simulink model "RainSnsrWiperMot_Method_2"  (R2021b)
settings: Solver=FixedStepDiscrete  StartTime=0.0  StopTime=20  FixedStep=0.01  RelTol=1e-3
model workspace (MAT data in the model file):
  Table_x_data = Simulink.Parameter
  Table_x_data.Value = [0 1 2 3 4 5 6 7]
  Table_x_data.DataType = 'auto'
  Table_x_data.Complexity = 'real'
  Table_x_data.Dimensions = [1 8]
  Table_y_data = Simulink.Parameter
  Table_y_data.Value = [0 0.4 0.45 0.5 0.55 0.6 0.65 0.7]
  Table_y_data.DataType = 'auto'
  Table_y_data.Complexity = 'real'
  Table_y_data.Dimensions = [1 8]
undefined symbols (not defined in the file or in its folder): sigbuilder_block
libraries: simulink x2
settings Model: Creator=waleed.elshemy  LastModifiedBy=waleed.elshemy
settings OptimizationCC: DefaultParameterBehavior=Inlined  UseDivisionForNetSlopeComputation=on  GainParamInheritBuiltInType=on  UseFloatMulNetSlope=on  InlineInvariantSignals=on  PassReuseOutputArgsAs=Individual arguments  ZeroExternalMemoryAtStartup=off  ZeroInternalMemoryAtStartup=off  NoFixptDivByZeroProtection=on  EfficientFloat2IntCast=on  LifeSpan=1  OptimizeBlockOrder=speed  DifferentSizesBufferReuse=on  EfficientTunableParamExpr=on
settings DebuggingCC: ParameterTunabilityLossMsg=error
settings HardwareCC: ProdLongLongMode=on
settings SFSimCC: MATLABDynamicMemAlloc=off
settings RTWCC: Description=Embedded Coder  SystemTargetFile=ert.tlc  TemplateMakefile=ert_default_tmf
settings CodeAppCC: ForceParamTrailComments=on  IgnoreCustomStorageClasses=off  OperatorAnnotations=on  SimulinkDataObjDesc=on  SFDataObjDesc=on  CustomSymbolStrGlobalVar=rt$N$M  CustomSymbolStrType=$N$M  CustomSymbolStrFcn=$N$M$F  CustomSymbolStrMacro=$N$M  InsertBlockDesc=on
settings ERTTargetCC: TargetLangStandard=C99 (ISO)  GenerateSampleERTMain=on  IncludeMdlTerminateFcn=off  CombineSignalStateStructs=on  SupportComplex=off  SupportNonInlinedSFcns=on  InlinedParameterPlacement=NonHierarchical  ERTCustomFileTemplate=example_file_process.tlc  ERTFilePackagingFormat=CompactWithDataFile

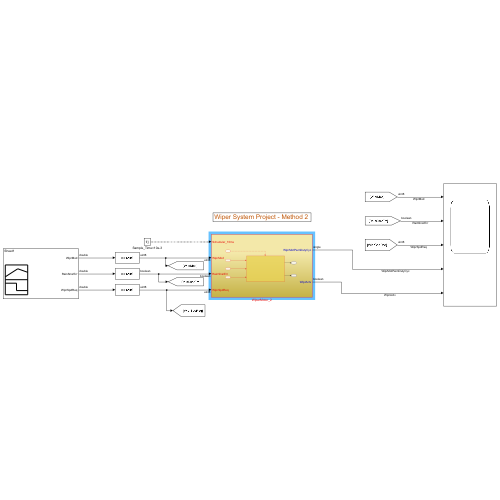
[thumbnail: Simulink's stored preview of the top-level diagram]
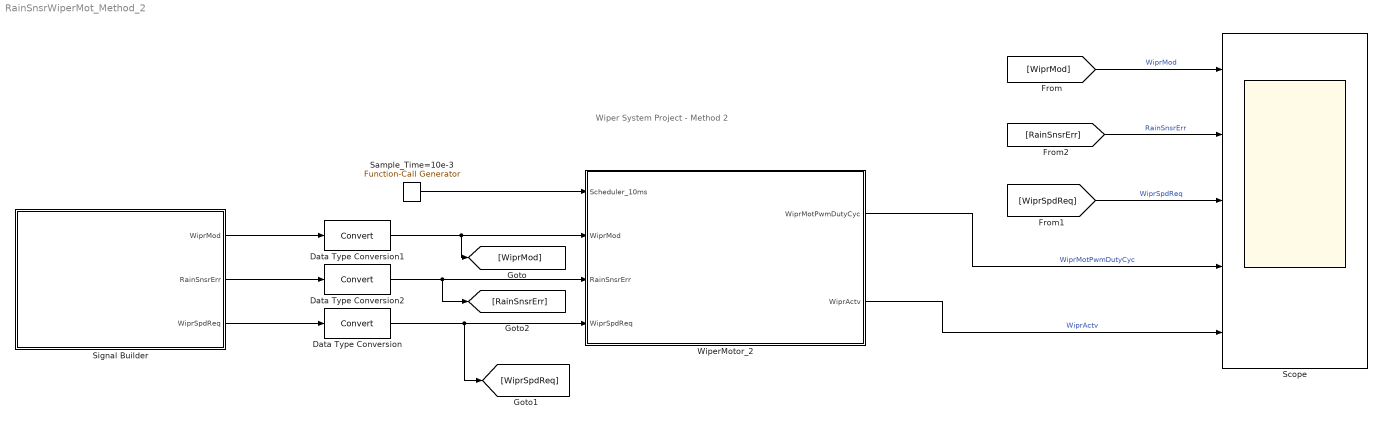
== system RainSnsrWiperMot_Method_2 ==
  note: Wiper System Project - Method 2
  Data Type Conversion : DataTypeConversion
  Data Type Conversion1 : DataTypeConversion
  Data Type Conversion2 : DataTypeConversion
  Sample_Time=10e-3 : simulink/Ports & Subsystems/Function-Call Generator  sample_time=0.01  numberOfIterations=1  DisallowWideOutput=off
  Scope : Scope  NumInputPorts=5
  Signal Builder : Subsystem  Tag=STV Subsys  LoadFcn=sigbuilder_block('load');  StartFcn=sigbuilder_block('start');  StopFcn=sigbuilder_block('stop');  ClipboardFcn=sigbuilder_block('clipboard');  mask(Sigbuilder block){tuvar=[0:10]}
      mask help: Simulink:masks:SigbuilderBlock_MD
      mask init:
      | if ~strcmp(get_param(bdroot(gcbh),'SimulationStatus'),'stopped') tuvar = sigbuilder_block('maskInit'); end
      settings: CopyFcn=sigbuilder_block('copy');  DeleteFcn=sigbuilder_block('delete');  ModelCloseFcn=sigbuilder_block('modelClose');  PreSaveFcn=sigbuilder_block('preSave');  PauseFcn=sigbuilder_block('pause');  ContinueFcn=sigbuilder_block('continue');  NameChangeFcn=sigbuilder_block('namechange');  OpenFcn=sigbuilder_block('open',[240 92.5 550.5 362.5 ]);  CloseFcn=sigbuilder_block('close');
      mask Display: plot(0, 0, 100, 100,[2, 2, 32, 32, 2], [68, 8, 8, 68, 68],[32, 2], [38, 38], [32, 19, 2],[53, 60, 44], [32, 17, 17, 2],[16, 16, 31, 31]);txt = getActiveGroup(gcbh);text(2, 100, txt,'verticalAlignment', 'top');
  WiperMotor_2 : Subsystem
  wires:
  Sample_Time=10e-3/1 -> WiperMotor_2/1(Scheduler_10ms)
  WiperMotor_2/1(WiprMotPwmDutyCyc) -> Scope/4  "WiprMotPwmDutyCyc"
  WiperMotor_2/2(WiprActv) -> Scope/5  "WiprActv"
  Signal Builder/1(WiprMod) -> Data Type Conversion1/1
  Signal Builder/2(RainSnsrErr) -> Data Type Conversion2/1
  Signal Builder/3(WiprSpdReq) -> Data Type Conversion/1
  Data Type Conversion/1 -> WiperMotor_2/4(WiprSpdReq), [WiprSpdReq]
  Data Type Conversion1/1 -> WiperMotor_2/2(WiprMod), [WiprMod]
  [WiprMod] -> Scope/1  "WiprMod"
  [WiprSpdReq] -> Scope/3  "WiprSpdReq"
  [RainSnsrErr] -> Scope/2  "RainSnsrErr"
  Data Type Conversion2/1 -> [RainSnsrErr], WiperMotor_2/3(RainSnsrErr)

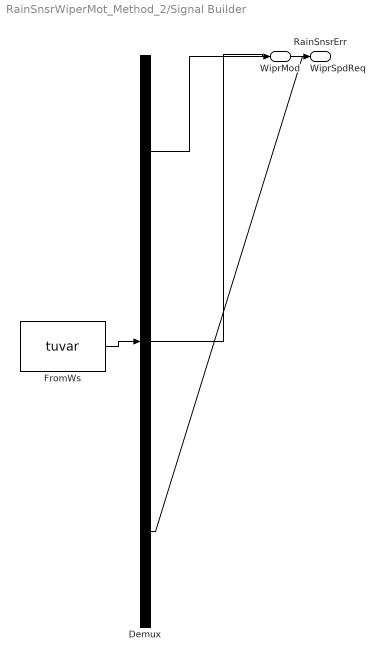
== system RainSnsrWiperMot_Method_2/Signal Builder ==
  Demux : Demux  Tag=STV Demux  Outputs=3
      settings: DisplayOption=none
  FromWs : FromWorkspace  Tag=STV FromWs  VariableName=tuvar  SampleTime=1  OutputAfterFinalValue=Holding final value
      SigBuilderData=|
      | common.afterFinalStr = 'Hold final value'
      | common.sampleTime = '1'
      | dataSet.timeRange = [0 16]
      | dataSet.name = 'Sheet1'
      | sbobj.Groups.Name = 'Sheet1'
      | sbobj.Groups.Signals(1).Name = 'WiprMod'
      | sbobj.Groups.Signals(1).XData = [0 1 2 3 4 5 6 7 8 9 10 11 12 13 14 15 16]
      | sbobj.Groups.Signals(1).YData = [0 0 2 2 3 3 1 1 1 1 1 1 1 1 1 1 1]
      | sbobj.Groups.Signals(2).Name = 'RainSnsrErr'
      | sbobj.Groups.Signals(2).XData = [0 1 2 3 4 5 6 7 8 9 10 11 12 13 14 15 16]
      | sbobj.Groups.Signals(2).YData = [0 0 0 0 0 0 0 0 0 0 0 0 0 0 0 1 0]
      | sbobj.Groups.Signals(3).Name = 'WiprSpdReq'
      | sbobj.Groups.Signals(3).XData = [0 1 2 3 4 5 6 7 8 9 10 11 12 13 14 15 16]
      | sbobj.Groups.Signals(3).YData = [0 0 0 0 0 0 0 0 1 2 3 4 5 6 7 7 7]
      | sbobj.Groups.TimeRange = [0 16]
  WiprMod : Outport  Tag=STV Outport
  RainSnsrErr : Outport  Tag=STV Outport  Port=2
  WiprSpdReq : Outport  Tag=STV Outport  Port=3
  wires:
  Demux/1 -> WiprMod/1
  FromWs/1 -> Demux/1
  Demux/2 -> RainSnsrErr/1
  Demux/3 -> WiprSpdReq/1

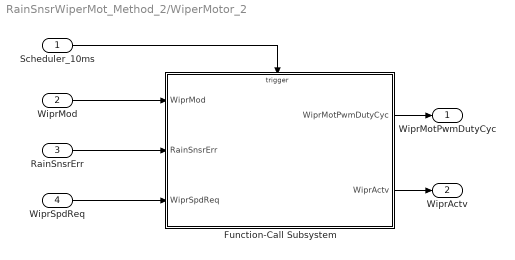
== system RainSnsrWiperMot_Method_2/WiperMotor_2 ==
  Scheduler_10ms : Inport
  WiprMod : Inport  Port=2  OutMin=0  OutMax=3  OutDataTypeStr=uint8
  RainSnsrErr : Inport  Port=3  OutMin=0  OutMax=1  OutDataTypeStr=boolean
  WiprSpdReq : Inport  Port=4  OutMin=0  OutMax=7  OutDataTypeStr=uint8
  Function-Call Subsystem : Subsystem  TreatAsAtomicUnit=on
  WiprMotPwmDutyCyc : Outport  OutMin=0  OutMax=1  OutDataTypeStr=single  LockScale=on
  WiprActv : Outport  Port=2  OutDataTypeStr=boolean
  wires:
  WiprMod/1 -> Function-Call Subsystem/1(WiprMod)
  WiprSpdReq/1 -> Function-Call Subsystem/3(WiprSpdReq)
  Function-Call Subsystem/2(WiprActv) -> WiprActv/1
  Scheduler_10ms/1 -> Function-Call Subsystem/Trigger
  RainSnsrErr/1 -> Function-Call Subsystem/2(RainSnsrErr)
  Function-Call Subsystem/1(WiprMotPwmDutyCyc) -> WiprMotPwmDutyCyc/1

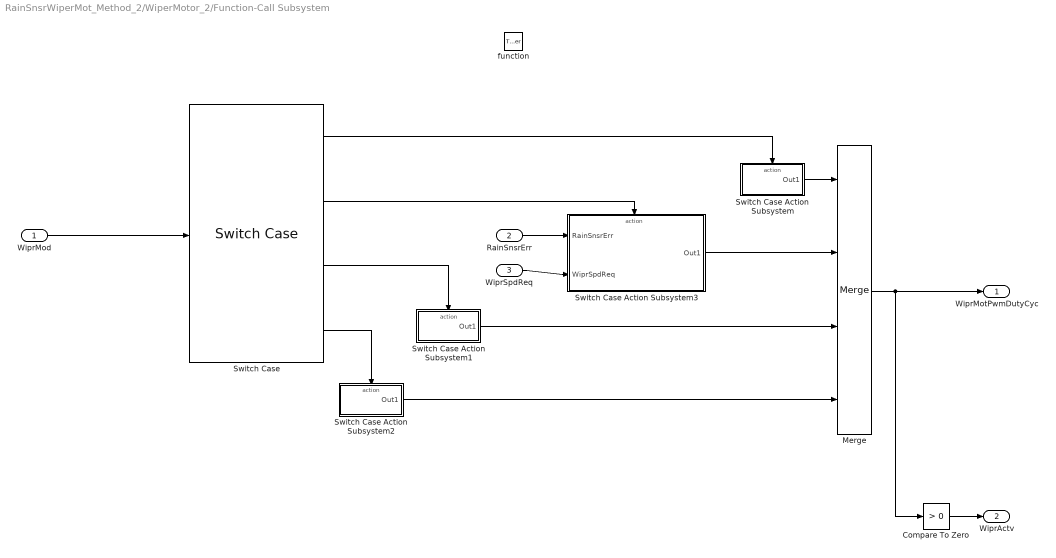
== system RainSnsrWiperMot_Method_2/WiperMotor_2/Function-Call Subsystem ==
  WiprMod : Inport
  RainSnsrErr : Inport  Port=2
  WiprSpdReq : Inport  Port=3
  function : TriggerPort  TriggerType=function-call  VariantControl=(inherit)
  Compare To Zero : simulink/Logic and Bit Operations/Compare To Zero  relop=>  OutDataTypeStr=boolean
  Merge : Merge  Inputs=4
  Switch Case : SwitchCase  CaseConditions={0,1,2,3}  ShowDefaultCase=off
  Switch Case Action Subsystem : Subsystem  TreatAsAtomicUnit=on
  Switch Case Action Subsystem1 : Subsystem  TreatAsAtomicUnit=on
  Switch Case Action Subsystem2 : Subsystem  TreatAsAtomicUnit=on
  Switch Case Action Subsystem3 : Subsystem  TreatAsAtomicUnit=on
  WiprMotPwmDutyCyc : Outport
  WiprActv : Outport  Port=2
  wires:
  WiprMod/1 -> Switch Case/1
  Switch Case/4 -> Switch Case Action Subsystem2/Action
  Switch Case/1 -> Switch Case Action Subsystem/Action
  Switch Case/2 -> Switch Case Action Subsystem3/Action
  Switch Case/3 -> Switch Case Action Subsystem1/Action
  Switch Case Action Subsystem/1(Out1) -> Merge/1
  Switch Case Action Subsystem3/1(Out1) -> Merge/2
  Switch Case Action Subsystem1/1(Out1) -> Merge/3
  Switch Case Action Subsystem2/1(Out1) -> Merge/4
  RainSnsrErr/1 -> Switch Case Action Subsystem3/1(RainSnsrErr)
  WiprSpdReq/1 -> Switch Case Action Subsystem3/2(WiprSpdReq)
  Merge/1 -> Compare To Zero/1, WiprMotPwmDutyCyc/1
  Compare To Zero/1 -> WiprActv/1

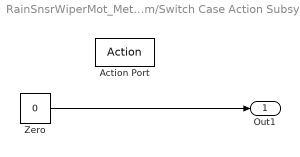
== system RainSnsrWiperMot_Method_2/WiperMotor_2/Function-Call Subsystem/Switch Case Action Subsystem ==
  Action Port : ActionPort  ActionPortLabel=case [ 0 ]:
  Zero : Constant  Value=0  OutDataTypeStr=Inherit: Inherit via back propagation
  Out1 : Outport
  wires:
  Zero/1 -> Out1/1

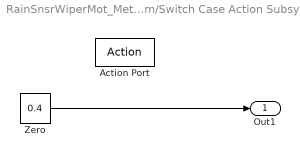
== system RainSnsrWiperMot_Method_2/WiperMotor_2/Function-Call Subsystem/Switch Case Action Subsystem1 ==
  Action Port : ActionPort  ActionPortLabel=case [ 2 ]:
  Zero : Constant  Value=0.4  OutDataTypeStr=single
  Out1 : Outport
  wires:
  Zero/1 -> Out1/1

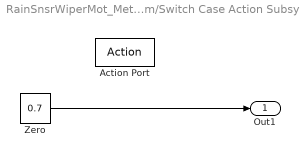
== system RainSnsrWiperMot_Method_2/WiperMotor_2/Function-Call Subsystem/Switch Case Action Subsystem2 ==
  Action Port : ActionPort  ActionPortLabel=case [ 3 ]:
  Zero : Constant  Value=0.7  OutDataTypeStr=Inherit: Inherit via back propagation
  Out1 : Outport
  wires:
  Zero/1 -> Out1/1

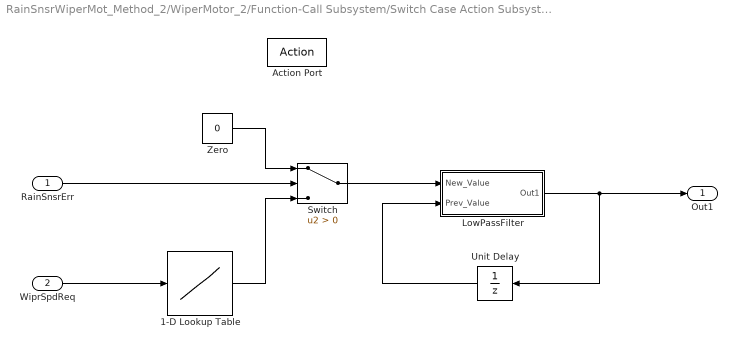
== system RainSnsrWiperMot_Method_2/WiperMotor_2/Function-Call Subsystem/Switch Case Action Subsystem3 ==
  RainSnsrErr : Inport
  WiprSpdReq : Inport  Port=2
  Action Port : ActionPort  ActionPortLabel=case [ 1 ]:
  1-D Lookup Table : Lookup_n-D  NumberOfTableDimensions=1  BreakpointsForDimension1=Table_x_data  Table=Table_y_data  TableDataTypeStr=single  ExtrapMethod=Clip  InternalRulePriority=Speed  OutDataTypeStr=single  RndMeth=Simplest  InputSameDT=on
  LowPassFilter : Subsystem
  Switch : Switch  Criteria=u2 > Threshold
  Unit Delay : UnitDelay  SampleTime=-1  HasFrameUpgradeWarning=on
  Zero : Constant  Value=0  OutDataTypeStr=Inherit: Inherit via back propagation
  Out1 : Outport
  wires:
  RainSnsrErr/1 -> Switch/2
  Zero/1 -> Switch/1
  WiprSpdReq/1 -> 1-D Lookup Table/1
  1-D Lookup Table/1 -> Switch/3
  Switch/1 -> LowPassFilter/1(New_Value)
  Unit Delay/1 -> LowPassFilter/2(Prev_Value)
  LowPassFilter/1(Out1) -> Out1/1, Unit Delay/1

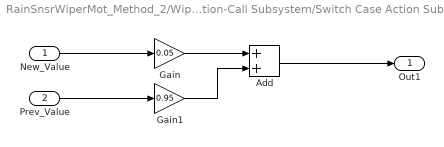
== system RainSnsrWiperMot_Method_2/WiperMotor_2/Function-Call Subsystem/Switch Case Action Subsystem3/LowPassFilter ==
  New_Value : Inport
  Prev_Value : Inport  Port=2
  Add : Sum
  Gain : Gain  Gain=0.05
  Gain1 : Gain  Gain=0.95
  Out1 : Outport
  wires:
  New_Value/1 -> Gain/1
  Prev_Value/1 -> Gain1/1
  Gain/1 -> Add/1
  Gain1/1 -> Add/2
  Add/1 -> Out1/1
